simulink model "demo_env"  (R2024a)
settings: Solver=FixedStepAuto  StartTime=0.0  StopTime=10.0  FixedStep=0.05  RelTol=1e-3
PostLoadFcn:
  | on_model_load
InitFcn:
  | on_model_start
StopFcn:
  | on_simulation_done
undefined symbols (not defined in the file or in its folder): ActiveScenario
libraries: demo_lib_ctl x2, demo_lib_sys x2
PostSaveFcn:
  | on_model_save
settings Model: Creator=luka  LastModifiedBy=luka

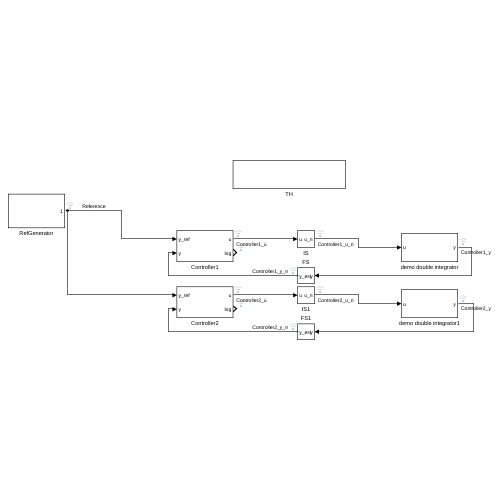
[thumbnail: Simulink's stored preview of the top-level diagram]
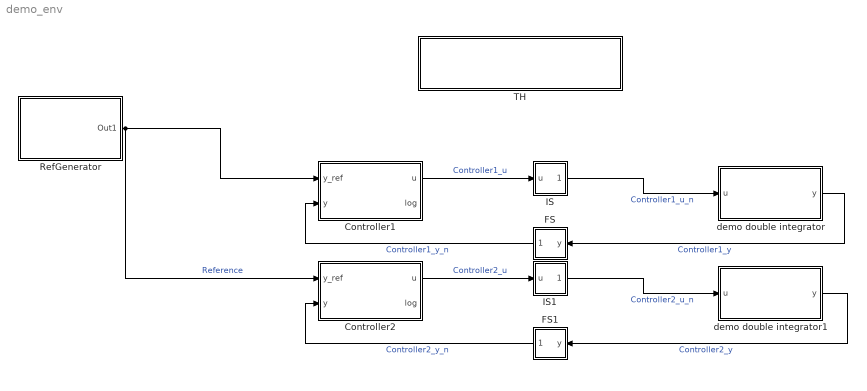
== system demo_env ==
  Controller1 : Subsystem
      mask DialogControl ParameterGroupVar Prompt: Params
  Controller2 : Subsystem
      mask DialogControl ParameterGroupVar Prompt: Params
  FS : Subsystem
  FS1 : Subsystem
  IS : Subsystem
  IS1 : Subsystem
  RefGenerator : Subsystem  mask{scenario=P1}
      settings: OpenFcn=on_reference_generator_open();
      mask TypeOptions scenario: P1
      mask Callback scenario: on_scenario_select;
  TH : Subsystem
      mask DialogControl ParameterGroupVar Prompt: Params
  demo double integrator : Subsystem
      mask DialogControl ParameterGroupVar Prompt: Params
  demo double integrator1 : Subsystem
      mask DialogControl ParameterGroupVar Prompt: Params
  wires:
  Controller1/1(u) -> IS/1(u)  "Controller1_u"
  IS/1(u_n) -> demo double integrator/1(u)  "Controller1_u_n"
  demo double integrator/1(y) -> FS/1(y)  "Controller1_y"
  FS/1(y_est) -> Controller1/2(y)  "Controller1_y_n"
  RefGenerator/1(Out1) -> Controller1/1(y_ref), Controller2/1(y_ref)  "Reference"
  Controller2/1(u) -> IS1/1(u)  "Controller2_u"
  IS1/1(u_n) -> demo double integrator1/1(u)  "Controller2_u_n"
  demo double integrator1/1(y) -> FS1/1(y)  "Controller2_y"
  FS1/1(y_est) -> Controller2/2(y)  "Controller2_y_n"

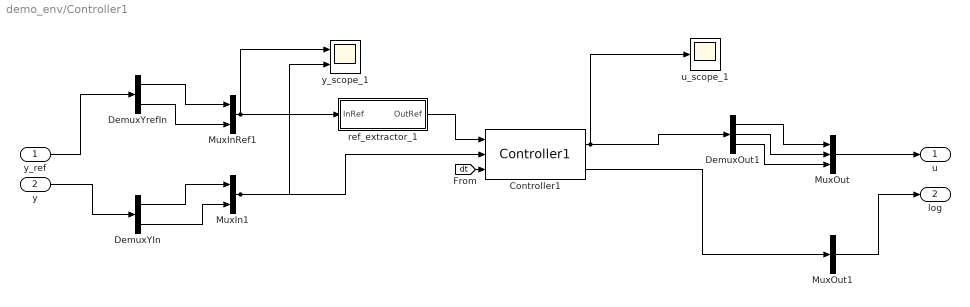
== system demo_env/Controller1 ==
  y_ref : Inport  PortDimensions=2
  y : Inport  Port=2  PortDimensions=2
  Controller1 : demo_lib_ctl/Controller1  Tag=__cs_comptype:ctl;__cs_compimpl:mat;  iid__=[50 100 51 56 48 99 57 99 45 101 56 53 53 45 52 53 55 51 45 56 98 48 57 45 49 97 54 102 50 100 57 52 51 54 102 97]  pid__=[67 111 110 116 114 111 108 108 101 114 49 58 100 101 109 111 95 108 105 98]  params=demo_env_params.ctl.Controller1  LogEntryType=Controller1_LT  data=Controller1_data  ParamsType=Controller1_PT  DataType=Controller1_DT  u_ic=0
  DemuxOut1 : Demux  Outputs=3
  DemuxYIn : Demux  Outputs=2
  DemuxYrefIn : Demux  Outputs=2
  MuxIn1 : Mux  Inputs=2
  MuxInRef1 : Mux  Inputs=2
  MuxOut : Mux  Inputs=3
  MuxOut1 : BusCreator  Inputs=1
  ref_extractor_1 : Subsystem
  u_scope_1 : Scope
  y_scope_1 : Scope  NumInputPorts=2
  u : Outport  PortDimensions=3
  log : Outport  Port=2
  wires:
  [dt] -> Controller1/3
  y/1 -> DemuxYIn/1
  y_ref/1 -> DemuxYrefIn/1
  MuxOut/1 -> u/1
  MuxOut1/1 -> log/1
  MuxInRef1/1 -> ref_extractor_1/1(InRef), y_scope_1/1
  ref_extractor_1/1(OutRef) -> Controller1/1
  MuxIn1/1 -> Controller1/2, y_scope_1/2
  Controller1/1 -> DemuxOut1/1, u_scope_1/1
  Controller1/2 -> MuxOut1/1
  DemuxYIn/1 -> MuxIn1/1
  DemuxYrefIn/1 -> MuxInRef1/1
  DemuxYIn/2 -> MuxIn1/2
  DemuxYrefIn/2 -> MuxInRef1/2
  DemuxOut1/1 -> MuxOut/1
  DemuxOut1/2 -> MuxOut/2
  DemuxOut1/3 -> MuxOut/3

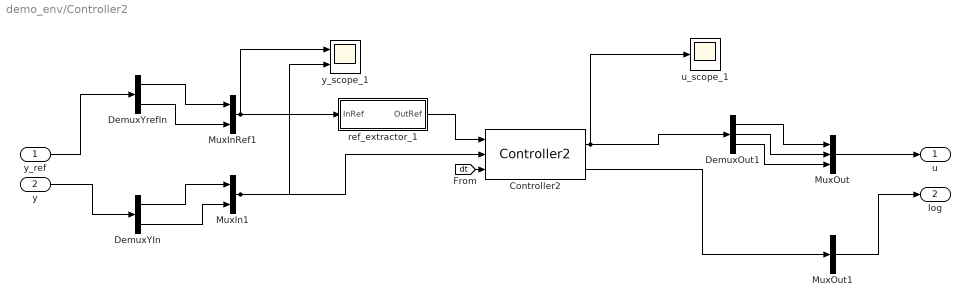
== system demo_env/Controller2 ==
  y_ref : Inport  PortDimensions=2
  y : Inport  Port=2  PortDimensions=2
  Controller2 : demo_lib_ctl/Controller2  Tag=__cs_comptype:ctl;__cs_compimpl:py;  iid__=[100 51 48 50 55 49 56 53 45 48 55 53 48 45 52 52 102 98 45 57 50 51 97 45 53 55 54 52 49 100 53 50 99 56 100 56]  pid__=[67 111 110 116 114 111 108 108 101 114 50 58 100 101 109 111 95 108 105 98]  params=demo_env_params.ctl.Controller2  LogEntryType=Controller2_LT  data=Controller2_data  DataType=Controller2_DT  u_ic=0
  DemuxOut1 : Demux  Outputs=3
  DemuxYIn : Demux  Outputs=2
  DemuxYrefIn : Demux  Outputs=2
  MuxIn1 : Mux  Inputs=2
  MuxInRef1 : Mux  Inputs=2
  MuxOut : Mux  Inputs=3
  MuxOut1 : BusCreator  Inputs=1
  ref_extractor_1 : Subsystem
  u_scope_1 : Scope
  y_scope_1 : Scope  NumInputPorts=2
  u : Outport  PortDimensions=3
  log : Outport  Port=2
  wires:
  [dt] -> Controller2/3
  y/1 -> DemuxYIn/1
  y_ref/1 -> DemuxYrefIn/1
  MuxOut/1 -> u/1
  MuxOut1/1 -> log/1
  MuxInRef1/1 -> ref_extractor_1/1(InRef), y_scope_1/1
  ref_extractor_1/1(OutRef) -> Controller2/1
  MuxIn1/1 -> Controller2/2, y_scope_1/2
  Controller2/1 -> DemuxOut1/1, u_scope_1/1
  Controller2/2 -> MuxOut1/1
  DemuxYIn/1 -> MuxIn1/1
  DemuxYrefIn/1 -> MuxInRef1/1
  DemuxYIn/2 -> MuxIn1/2
  DemuxYrefIn/2 -> MuxInRef1/2
  DemuxOut1/1 -> MuxOut/1
  DemuxOut1/2 -> MuxOut/2
  DemuxOut1/3 -> MuxOut/3

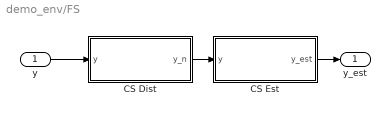
== system demo_env/FS ==
  y : Inport
  CS Dist : Subsystem
      mask DialogControl ParameterGroupVar Prompt: Params
  CS Est : Subsystem
      mask DialogControl ParameterGroupVar Prompt: Params
  y_est : Outport
  wires:
  CS Est/1(y_est) -> y_est/1
  CS Dist/1(y_n) -> CS Est/1(y)
  y/1 -> CS Dist/1(y)

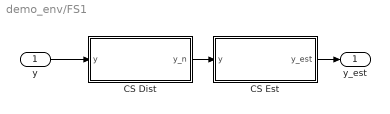
== system demo_env/FS1 ==
  y : Inport
  CS Dist : Subsystem
      mask DialogControl ParameterGroupVar Prompt: Params
  CS Est : Subsystem
      mask DialogControl ParameterGroupVar Prompt: Params
  y_est : Outport
  wires:
  CS Est/1(y_est) -> y_est/1
  CS Dist/1(y_n) -> CS Est/1(y)
  y/1 -> CS Dist/1(y)

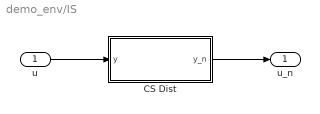
== system demo_env/IS ==
  u : Inport
  CS Dist : Subsystem
      mask DialogControl ParameterGroupVar Prompt: Params
  u_n : Outport
  wires:
  CS Dist/1(y_n) -> u_n/1
  u/1 -> CS Dist/1(y)

== system demo_env/IS1 ==
  u : Inport
  CS Dist : Subsystem
      mask DialogControl ParameterGroupVar Prompt: Params
  u_n : Outport
  wires:
  CS Dist/1(y_n) -> u_n/1
  u/1 -> CS Dist/1(y)

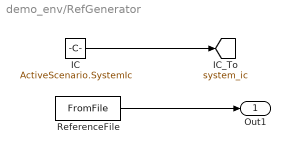
== system demo_env/RefGenerator ==
  IC : Constant  Value=ActiveScenario.SystemIc
  ReferenceFile : FromFile  SampleTime=0
  Out1 : Outport
  tag scope: system_ic=global
  wires:
  IC/1 -> [system_ic]
  ReferenceFile/1 -> Out1/1

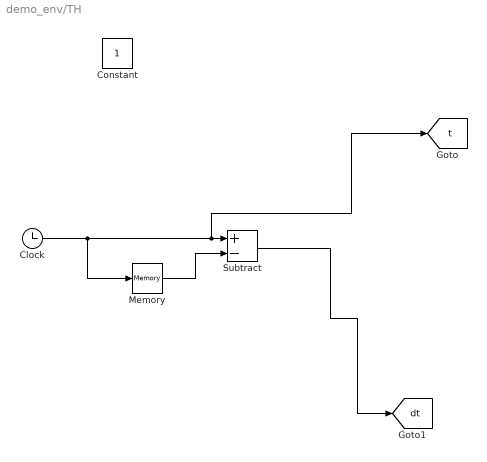
== system demo_env/TH ==
  Clock : Clock
  Constant : Constant
  Memory : Memory
  Subtract : Sum  Inputs=+-
  tag scope: dt=global, t=global
  wires:
  Subtract/1 -> [dt]
  Memory/1 -> Subtract/2
  Clock/1 -> Memory/1, Subtract/1, [t]

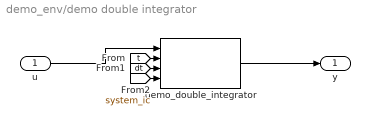
== system demo_env/demo double integrator ==
  u : Inport
  demo_double_integrator : demo_lib_sys/demo_double_integrator  Tag=__cs_comptype:sys;__cs_compimpl:slx;  k1=0  k2=0  iid__=[56 52 101 51 97 57 97 52 45 51 97 97 54 45 52 49 49 52 45 98 100 98 51 45 52 48 54 100 48 97 98 49 51 98 56 100]  pid__=[100 101 109 111 95 100 111 117 98 108 101 95 105 110 116 101 103 114 97 116 111 114 58 100 101 109 111 95 108 105 98]  params=ActiveScenario.SystemParams  params_struct_name=demo_env_params.sys.demoDoubleIntegrator
  y : Outport
  wires:
  u/1 -> demo_double_integrator/1
  demo_double_integrator/1 -> y/1
  [t] -> demo_double_integrator/2
  [dt] -> demo_double_integrator/3
  [system_ic] -> demo_double_integrator/4

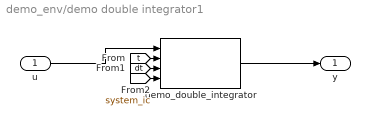
== system demo_env/demo double integrator1 ==
  u : Inport
  demo_double_integrator : demo_lib_sys/demo_double_integrator  Tag=__cs_comptype:sys;__cs_compimpl:slx;  k1=0  k2=0  iid__=[56 52 101 51 97 57 97 52 45 51 97 97 54 45 52 49 49 52 45 98 100 98 51 45 52 48 54 100 48 97 98 49 51 98 56 100]  pid__=[100 101 109 111 95 100 111 117 98 108 101 95 105 110 116 101 103 114 97 116 111 114 58 100 101 109 111 95 108 105 98]  params=ActiveScenario.SystemParams  params_struct_name=demo_env_params.sys.demoDoubleIntegrator
  y : Outport
  wires:
  u/1 -> demo_double_integrator/1
  demo_double_integrator/1 -> y/1
  [t] -> demo_double_integrator/2
  [dt] -> demo_double_integrator/3
  [system_ic] -> demo_double_integrator/4

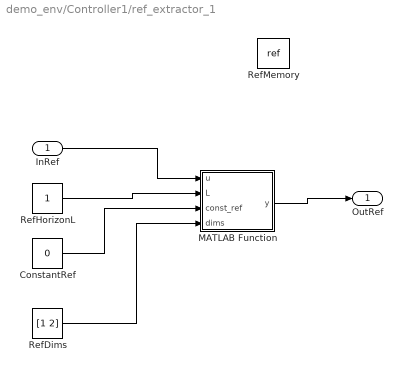
== system demo_env/Controller1/ref_extractor_1 ==
  InRef : Inport
  ConstantRef : Constant  Value=0
  MATLAB Function : MATLAB Function  TreatAsAtomicUnit=on
  RefDims : Constant  Value=[1 2]
  RefHorizonL : Constant
  RefMemory : DataStoreMemory  DataStoreName=ref  WriteAfterWriteMsg=warning  ShowAdditionalParam=off  OutDataTypeStr=double
  OutRef : Outport
  wires:
  ConstantRef/1 -> MATLAB Function/3(const_ref)
  RefDims/1 -> MATLAB Function/4(dims)
  RefHorizonL/1 -> MATLAB Function/2(L)
  InRef/1 -> MATLAB Function/1(u)
  MATLAB Function/1(y) -> OutRef/1

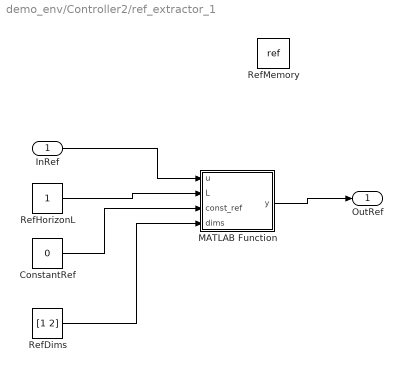
== system demo_env/Controller2/ref_extractor_1 ==
  InRef : Inport
  ConstantRef : Constant  Value=0
  MATLAB Function : MATLAB Function  TreatAsAtomicUnit=on
  RefDims : Constant  Value=[1 2]
  RefHorizonL : Constant
  RefMemory : DataStoreMemory  DataStoreName=ref  WriteAfterWriteMsg=warning  ShowAdditionalParam=off  OutDataTypeStr=double
  OutRef : Outport
  wires:
  ConstantRef/1 -> MATLAB Function/3(const_ref)
  RefDims/1 -> MATLAB Function/4(dims)
  RefHorizonL/1 -> MATLAB Function/2(L)
  InRef/1 -> MATLAB Function/1(u)
  MATLAB Function/1(y) -> OutRef/1

== system demo_env/FS/CS Dist ==
  y : Inport
  Gain : Gain
  y_n : Outport
  wires:
  Gain/1 -> y_n/1
  y/1 -> Gain/1

== system demo_env/FS/CS Est ==
  y : Inport
  Gain : Gain
  y_est : Outport
  wires:
  y/1 -> Gain/1
  Gain/1 -> y_est/1

== system demo_env/FS1/CS Dist ==
  y : Inport
  Gain : Gain
  y_n : Outport
  wires:
  Gain/1 -> y_n/1
  y/1 -> Gain/1

== system demo_env/FS1/CS Est ==
  y : Inport
  Gain : Gain
  y_est : Outport
  wires:
  y/1 -> Gain/1
  Gain/1 -> y_est/1

== system demo_env/IS/CS Dist ==
  y : Inport
  Gain : Gain
  y_n : Outport
  wires:
  y/1 -> Gain/1
  Gain/1 -> y_n/1

== system demo_env/IS1/CS Dist ==
  y : Inport
  Gain : Gain
  y_n : Outport
  wires:
  y/1 -> Gain/1
  Gain/1 -> y_n/1

== matlab function demo_env/Controller2/ref_extractor_1/MATLAB Function ==
  settings: updateMethod=DISCRETE
  data: u input; L input; const_ref input; dims input; y output; ref data_store_memory; GlobalReference parameter
function y = fcn(u, L, const_ref, dims, GlobalReference)

persistent cnt
global ref

if isempty(cnt)
    cnt = 0;
end
cnt = cnt+1;

horizon_end = cnt+L-1;
if L > 1 
   if horizon_end > length(GlobalReference)
        if size(ref, 1) == size(u, 1)
            y = permute(ref, [2, 1]);
        else
            y = ref;
        end       
        return
   end

   if size(ref, 1) == size(u, 1)
      
      if const_ref == 0
        ref(:, :) = GlobalReference(cnt:horizon_end, dims)';
      else
        ref(:, :) = repmat(GlobalReference(cnt, dims)', 1, L);
      end
      y = permute(ref, [2, 1]);
   else
      if const_ref == 0
        ref(1:L, :) = GlobalReference(cnt:horizon_end, dims);
      else
        ref(1:L, :) = repmat(GlobalReference(cnt, dims), L, 1);
      end
      y = ref;
   end
else
   if size(ref, 1) == size(u, 1)
       ref = u;
       y = permute(ref, [2, 1]);
   else
      ref(1, :) = u';
      y = ref;
   end
end

== matlab function demo_env/Controller1/ref_extractor_1/MATLAB Function ==
  settings: updateMethod=DISCRETE
  data: u input; L input; const_ref input; dims input; y output; ref data_store_memory; GlobalReference parameter
function y = fcn(u, L, const_ref, dims, GlobalReference)

persistent cnt
global ref

if isempty(cnt)
    cnt = 0;
end
cnt = cnt+1;

horizon_end = cnt+L-1;
if L > 1 
   if horizon_end > length(GlobalReference)
        if size(ref, 1) == size(u, 1)
            y = permute(ref, [2, 1]);
        else
            y = ref;
        end       
        return
   end

   if size(ref, 1) == size(u, 1)
      
      if const_ref == 0
        ref(:, :) = GlobalReference(cnt:horizon_end, dims)';
      else
        ref(:, :) = repmat(GlobalReference(cnt, dims)', 1, L);
      end
      y = permute(ref, [2, 1]);
   else
      if const_ref == 0
        ref(1:L, :) = GlobalReference(cnt:horizon_end, dims);
      else
        ref(1:L, :) = repmat(GlobalReference(cnt, dims), L, 1);
      end
      y = ref;
   end
else
   if size(ref, 1) == size(u, 1)
       ref = u;
       y = permute(ref, [2, 1]);
   else
      ref(1, :) = u';
      y = ref;
   end
end
